simulink model "gm_hdlcoder_led_blinking"  (R2017a)
settings: Solver=FixedStepDiscrete  StartTime=0.0  StopTime=inf  RelTol=1e-3
InitFcn:
  | Ts = 1e-3;
libraries: simulink x2, hdlsllib x2
settings Model: Creator=wchen  LastModifiedBy=hyang344
settings DataIOCC: LimitDataPoints=on  SaveFormat=Array  SaveOutput=off  SignalLogging=off  SaveTime=off
settings OptimizationCC: BlockReduction=off  ConditionallyExecuteInputs=off  DefaultParameterBehavior=Inlined  ExpressionDepthLimit=2147483647  LifeSpan=inf
settings DebuggingCC: AlgebraicLoopMsg=error  UnderspecifiedInitializationDetection=Classic  MergeDetectMultiDrivingBlocksExec=none  SolverPrmCheckMsg=warning  InheritedTsInSrcMsg=none  SingleTaskRateTransMsg=error  ParameterPrecisionLossMsg=none  StateNameClashWarn=warning  SFUnexpectedBacktrackingDiag=warning  SFNoUnconditionalDefaultTransitionDiag=warning  SFExecutionAtInitializationDiag=none
settings HardwareCC: ProdBitPerPointer=32  ProdBitPerSizeT=32  ProdBitPerPtrDiffT=32  ProdLargestAtomicFloat=None  ProdIntDivRoundTo=Undefined  ProdEndianess=Unspecified  ProdWordSize=32  ProdHWDeviceType=ASIC/FPGA->ASIC/FPGA  ProdEqTarget=off
settings ModelReferenceCC: PropagateSignalLabelsOutOfModel=off
settings GRTTargetCC: TargetLangStandard=C89/C90 (ANSI)  GeneratePreprocessorConditionals=Disable all
settings ConfigComp: CovMetricSettings=dw  CovHtmlReporting=on  CovSaveCumulativeToWorkspaceVar=on  CovSaveSingleToWorkspaceVar=on  CovExternalEMLEnable=off

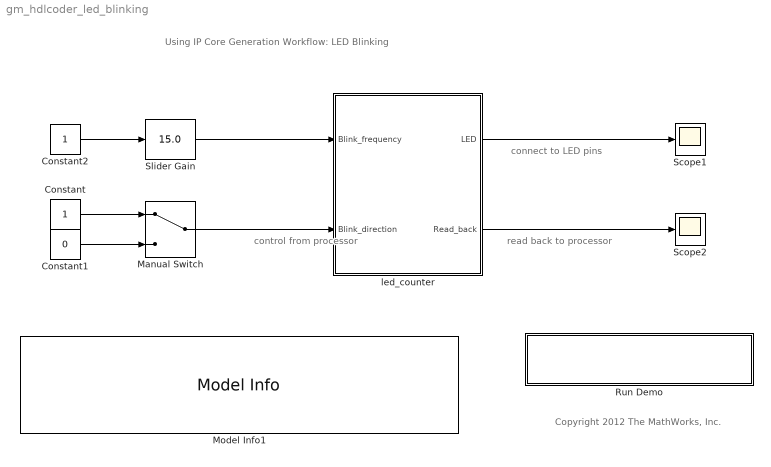
== system gm_hdlcoder_led_blinking ==
  note: read back to
      | processor
  note: connect to
      | LED pins
  note: control from
      | processor
  note: Using IP Core Generation Workflow: LED Blinking
  note: Copyright 2012 The MathWorks, Inc.
  Constant : Constant  OutDataTypeStr=boolean  SampleTime=Ts
  Constant1 : Constant  Value=0  OutDataTypeStr=boolean  SampleTime=Ts
  Constant2 : Constant  OutDataTypeStr=fixdt(0, 4, 0)  SampleTime=Ts
  Manual Switch : ManualSwitch
  Model Info1 : simulink/Model-Wide Utilities/Model Info  InitialBlockCM=None  BlockCM=None  Frame=on  DisplayStringWithTags=|  HorizontalTextAlignment=Left  LeftAlignmentValue=0.02  SourceBlockDiagram=hdlcoder_led_blinking  TagMaxNumber=20
      | This example shows how to use HDL Workflow Advisor to 
      | generate a custom IP core which blink LEDs on FPGA board.
      | 
      | In MATLAB, type the following:
      |   hdladvisor('hdlcoder_led_blinking/led_counter')
  Run Demo : Subsystem
      settings: OpenFcn=hdladvisor([bdroot, '/led_counter'])
      mask Display: disp('Launch HDL Workflow Advisor')
  Scope1 : Scope
  Scope2 : Scope
  Slider Gain : simulink/Math Operations/Slider Gain  gain=15.0  low=0  high=15
  led_counter : Subsystem  TreatAsAtomicUnit=on
  wires:
  led_counter/1(LED) -> Scope1/1
  led_counter/2(Read_back) -> Scope2/1
  Slider Gain/1 -> led_counter/1(Blink_frequency)
  Constant2/1 -> Slider Gain/1
  Manual Switch/1 -> led_counter/2(Blink_direction)
  Constant1/1 -> Manual Switch/2
  Constant/1 -> Manual Switch/1

== system gm_hdlcoder_led_blinking/Run Demo ==

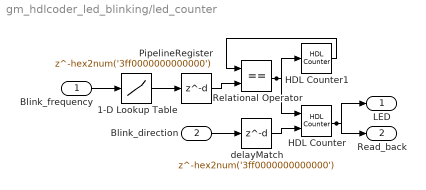
== system gm_hdlcoder_led_blinking/led_counter ==
  Blink_frequency : Inport  OutDataTypeStr=fixdt(0, 4, 0)  SampleTime=0.001
  Blink_direction : Inport  Port=2  OutDataTypeStr=boolean  SampleTime=0.001
  1-D Lookup Table : Lookup_n-D  NumberOfTableDimensions=1  BreakpointsForDimension1=[fi(0,0,4,0,'hex','0') fi(0,0,4,0,'hex','1') fi(0,0,4,0,'hex','2') fi(0,0,4,0,'hex','3') fi(0,0,4,0,'hex','4') fi(0,0,4,0,'hex','5') fi(0,0,4,0,'hex','6') fi(0,0,4,0,'hex','7') fi(0,0,4,0,'hex','8') fi(0,0,4,0,'hex','9') fi(0,0,4,0,'hex','a') fi(0,0,4,0,'hex','b') fi(0,0,4,0,'hex','c') fi(0,0,4,0,'hex','d') fi(0,0,4,0,'hex','e') fi(0,0,4,0,'hex','f')]  Table="reshape([fi(0,0,24,0,'hex','800000') fi(0,0,24,0,'hex','400000') fi(0,0,24,0,'hex','200000') fi(0,0,24,0,'hex','100000') fi(0,0,24,0,'hex','080000') fi(0,0,24,0,'hex','040000') fi(0,0,24,0,'hex','020000') fi(0,0,24,0,'hex','010000') fi(0,0,24,0,'hex','008000') fi(0,0,24,0,'hex','004000') fi(0,0,24,0,'hex','002000') fi(0,0,24,0,'hex','001000') fi(0,0,24,0,'hex','000800') fi(0,0,24,0,'hex','000400') fi(0,0,24,0,'hex','000200') fi(0,0,24,0,'hex','000100')].', [1  16])"  InterpMethod=Flat  DiagnosticForOutOfRangeInput=Error  SampleTime=0.001  OutDataTypeStr=fixdt(0, 24, 0)  RndMeth=Simplest  InputSameDT=on
  HDL Counter : hdlsllib/HDL Operations/HDL Counter  CountType=Free running  CountInit=hex2num('0000000000000000')  CountStep=hex2num('3ff0000000000000')  CountMax=25  CountFromType=Initial value  CountFrom=hex2num('0000000000000000')  CountResetPort=off  CountLoadPort=off  CountEnbPort=on  CountDirPort=on  CountDataType=Unsigned  CountWordLen=8  CountFracLen=0  CountSampTime=0.001
      settings: SourceProductName=HDL Coder  SourceProductBaseCode=HD
  HDL Counter1 : hdlsllib/HDL Operations/HDL Counter  CountType=Free running  CountInit=hex2num('0000000000000000')  CountStep=hex2num('3ff0000000000000')  CountMax=25  CountFromType=Initial value  CountFrom=hex2num('0000000000000000')  CountResetPort=on  CountLoadPort=off  CountEnbPort=off  CountDirPort=off  CountDataType=Unsigned  CountWordLen=24  CountFracLen=0  CountSampTime=0.001
      settings: SourceProductName=HDL Coder  SourceProductBaseCode=HD
  PipelineRegister : Delay  DelayLength=hex2num('3ff0000000000000')  InitialCondition=0  InputProcessing=Inherited  SampleTime=0.001
  Relational Operator : RelationalOperator  Operator===  OutDataTypeStr=boolean  SampleTime=0.001  RndMeth=Nearest
  delayMatch : Delay  DelayLength=hex2num('3ff0000000000000')  InitialCondition=0  InputProcessing=Inherited  SampleTime=0.001
  LED : Outport
  Read_back : Outport  Port=2
  wires:
  Blink_frequency/1 -> 1-D Lookup Table/1
  delayMatch/1 -> HDL Counter/2
  PipelineRegister/1 -> Relational Operator/2
  HDL Counter/1 -> Read_back/1, LED/1
  Blink_direction/1 -> delayMatch/1
  HDL Counter1/1 -> Relational Operator/1
  Relational Operator/1 -> HDL Counter1/1, HDL Counter/1
  1-D Lookup Table/1 -> PipelineRegister/1
